simulink model "SLWF"  (R2022b)
settings: configuration reference "CommonModelConfiguration" (kept outside this file)
undefined symbols (not defined in the file): cc_param_251, LCFG_ISA_Intervention_Timeout, LCFG_ISAReactivation, LCFG_ISASoundRequest, LCFG_SLWF_Deactivation_Timeout, LCFG_VehicleBrand
settings Model: Creator=JELIASS5  LastModifiedBy=OTHOMSO1
settings ConfigSetRef: SourceName=CommonModelConfiguration  SourceLocation=Base Workspace

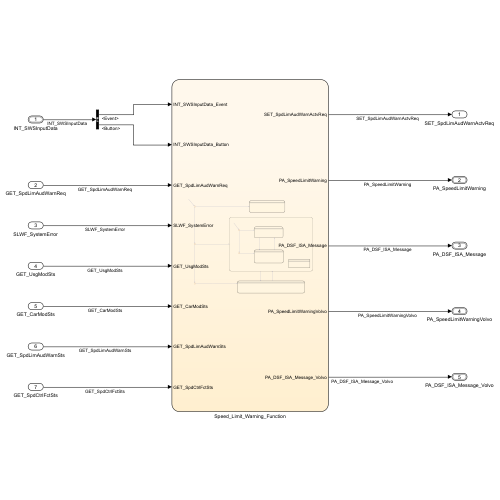
[thumbnail: Simulink's stored preview of the top-level diagram]
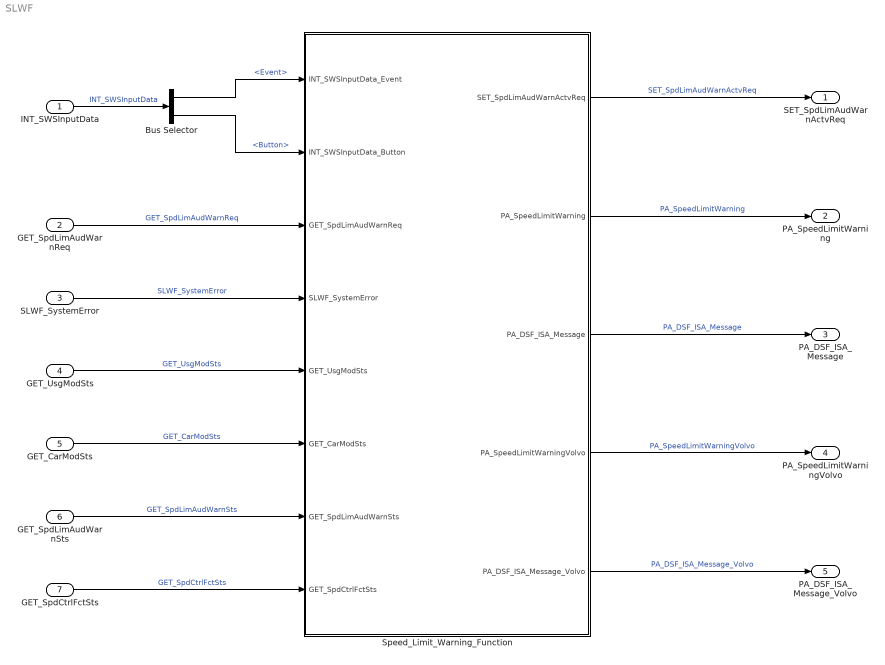
== system SLWF ==
  INT_SWSInputData : Inport  OutDataTypeStr=Bus: SWSInputData
  GET_SpdLimAudWarnReq : Inport  Port=2  OutDataTypeStr=Enum: OnOff1
  SLWF_SystemError : Inport  Port=3  OutDataTypeStr=boolean
  "GET_UsgModSts " : Inport  Port=4  OutDataTypeStr=Enum: UsgModSts1
  GET_CarModSts : Inport  Port=5  OutDataTypeStr=Enum: CarModSts1
  GET_SpdLimAudWarnSts : Inport  Port=6  OutDataTypeStr=Enum: WarnSts
  GET_SpdCtrlFctSts : Inport  Port=7  OutDataTypeStr=Enum: FctStsSpdCtrl
  Bus Selector : BusSelector  OutputSignals=Event,Button
  Speed_Limit_Warning_Function : Stateflow chart  TreatAsAtomicUnit=on
  SET_SpdLimAudWarnActvReq : Outport  OutDataTypeStr=Enum: OnOff1
  PA_SpeedLimitWarning : Outport  Port=2  OutDataTypeStr=Bus: PA_StatusAndWarningAndOffOnValue
  PA_DSF_ISA_Message : Outport  Port=3  OutDataTypeStr=Bus: PA_StatusAndOffOnValue
  PA_SpeedLimitWarningVolvo : Outport  Port=4  OutDataTypeStr=Bus: PA_StatusAndWarningAndOffOnValue
  PA_DSF_ISA_Message_Volvo : Outport  Port=5  OutDataTypeStr=Bus: PA_StatusAndOffOnValue
  wires:
  INT_SWSInputData/1 -> Bus Selector/1  "INT_SWSInputData"
  Bus Selector/1 -> Speed_Limit_Warning_Function/1(INT_SWSInputData_Event)  "<Event>"
  Bus Selector/2 -> Speed_Limit_Warning_Function/2(INT_SWSInputData_Button)  "<Button>"
  Speed_Limit_Warning_Function/1(SET_SpdLimAudWarnActvReq) -> SET_SpdLimAudWarnActvReq/1  "SET_SpdLimAudWarnActvReq"
  GET_SpdLimAudWarnReq/1 -> Speed_Limit_Warning_Function/3(GET_SpdLimAudWarnReq)  "GET_SpdLimAudWarnReq"
  Speed_Limit_Warning_Function/2(PA_SpeedLimitWarning) -> PA_SpeedLimitWarning/1  "PA_SpeedLimitWarning"
  SLWF_SystemError/1 -> Speed_Limit_Warning_Function/4(SLWF_SystemError)  "SLWF_SystemError"
  "GET_UsgModSts "/1 -> Speed_Limit_Warning_Function/5(GET_UsgModSts)  "GET_UsgModSts"
  GET_CarModSts/1 -> Speed_Limit_Warning_Function/6(GET_CarModSts)  "GET_CarModSts"
  GET_SpdLimAudWarnSts/1 -> Speed_Limit_Warning_Function/7(GET_SpdLimAudWarnSts)  "GET_SpdLimAudWarnSts"
  Speed_Limit_Warning_Function/3(PA_DSF_ISA_Message) -> PA_DSF_ISA_Message/1  "PA_DSF_ISA_Message"
  GET_SpdCtrlFctSts/1 -> Speed_Limit_Warning_Function/8(GET_SpdCtrlFctSts)  "GET_SpdCtrlFctSts"
  Speed_Limit_Warning_Function/4(PA_SpeedLimitWarningVolvo) -> PA_SpeedLimitWarningVolvo/1  "PA_SpeedLimitWarningVolvo"
  Speed_Limit_Warning_Function/5(PA_DSF_ISA_Message_Volvo) -> PA_DSF_ISA_Message_Volvo/1  "PA_DSF_ISA_Message_Volvo"

== stateflow chart SLWF/Speed_Limit_Warning_Function ==
  state CARCONFIG_INVALID
    en, du:
    SET_SpdLimAudWarnActvReq = OnOff1.OnOff1_Off;
    state CARCONFIG_INVALID_VOLVO
      en, du:
      PA_SpeedLimitWarningVolvo.Status = E_CommonStatus.NotPresent;
      PA_DSF_ISA_Message_Volvo.Status = E_CommonStatus.NotPresent;
      PA_SpeedLimitWarningVolvo.Value = E_OffOn.Off;
      PA_DSF_ISA_Message_Volvo.Value = E_OffOn.Off;
      PA_SpeedLimitWarningVolvo.Warning = E_OffOn.Off;
    state CARCONFIG_INVALID_POLESTAR
      en, du:
      PA_SpeedLimitWarning.Status = E_CommonStatus.NotPresent;
      PA_DSF_ISA_Message.Status = E_CommonStatus.NotPresent;
      PA_SpeedLimitWarning.Value = E_OffOn.Off;
      PA_DSF_ISA_Message.Value = E_OffOn.Off;
      PA_SpeedLimitWarning.Warning = E_OffOn.Off;
    (default) -> (junction 257)
    (junction 257) -> CARCONFIG_INVALID_VOLVO [order 2]
    (junction 257) -> CARCONFIG_INVALID_POLESTAR [order 1] : %Polestar
        | [LCFG_VehicleBrand == 2]
  state SYSTEM_OK
    state NOT_ACTIVE
      en, du:
      SET_SpdLimAudWarnActvReq = OnOff1.OnOff1_Off;
      state NOT_ACTIVE_VOLVO
        en, du:
        PA_SpeedLimitWarningVolvo.Status = E_CommonStatus.Disabled;
        PA_DSF_ISA_Message_Volvo.Status = E_CommonStatus.Disabled;
        PA_SpeedLimitWarningVolvo.Value = E_OffOn.Off;
        PA_DSF_ISA_Message_Volvo.Value = E_OffOn.Off;
        PA_SpeedLimitWarningVolvo.Warning = E_OffOn.Off;
      state NOT_ACTIVE_POLESTAR
        en, du:
        PA_SpeedLimitWarning.Status = E_CommonStatus.Disabled;
        PA_DSF_ISA_Message.Status = E_CommonStatus.Disabled;
        PA_SpeedLimitWarning.Value = E_OffOn.Off;
        PA_DSF_ISA_Message.Value = E_OffOn.Off;
        PA_SpeedLimitWarning.Warning = E_OffOn.Off;
      (default) -> (junction 251)
      (junction 251) -> NOT_ACTIVE_VOLVO [order 2]
      (junction 251) -> NOT_ACTIVE_POLESTAR [order 1] : %Polestar
          | [LCFG_VehicleBrand == 2]
    state ACTIVE
      state BUTTON_INTERACTION [parallel]
        settings: executionOrder=1
        state REQUEST_ON
          en, du: SET_SpdLimAudWarnActvReq = OnOff1.OnOff1_On;
        state REQUEST_OFF
          en, du: SET_SpdLimAudWarnActvReq = OnOff1.OnOff1_Off;
        (default) -> REQUEST_OFF
        REQUEST_OFF -> REQUEST_ON : %Button L2 pressed
            | [INT_SWSInputData_Button == E_SWSButton.BtnL2Req &&...
            | hasChangedTo(INT_SWSInputData_Event, E_SWSEvent.Push)]
        REQUEST_ON -> REQUEST_OFF : %Request times out
            | after(LCFG_ISASoundRequest, sec)
      state DSF_MESSAGES [parallel]
        settings: executionOrder=2
        state DSF_MESSAGE_VOLVO
          en, du:
          PA_SpeedLimitWarning.Status = E_CommonStatus.Disabled;
          PA_DSF_ISA_Message.Status = E_CommonStatus.Disabled;
          PA_SpeedLimitWarningVolvo.Status = E_CommonStatus.Available;
          PA_DSF_ISA_Message_Volvo.Status = E_CommonStatus.Available;
          state INTERVENTION
            en, du:
            PA_DSF_ISA_Message_Volvo.Value = E_OffOn.Off;
            PA_SpeedLimitWarningVolvo.Warning = E_OffOn.Off;
            PA_SpeedLimitWarningVolvo.Value = E_OffOn.On;
          state NO_MESSAGE
            en, du:
            PA_DSF_ISA_Message_Volvo.Value = E_OffOn.Off;
            PA_SpeedLimitWarningVolvo.Warning = E_OffOn.Off;
            PA_SpeedLimitWarningVolvo.Value = E_OffOn.Off;
          state MESSAGE_DISPLAYED
            en, du:
            PA_DSF_ISA_Message_Volvo.Value = E_OffOn.On;
            PA_SpeedLimitWarningVolvo.Warning = E_OffOn.On;
            PA_SpeedLimitWarningVolvo.Value = E_OffOn.Off;
          state WAIT
          state REACTIVATION_ICON
            en, du:
            PA_DSF_ISA_Message_Volvo.Value = E_OffOn.Off;
            PA_SpeedLimitWarningVolvo.Warning = E_OffOn.Off;
            PA_SpeedLimitWarningVolvo.Value = E_OffOn.On;
          (default) -> SYSTEM_OK.ACTIVE.DSF_MESSAGES.DSF_MESSAGE_VOLVO.NO_MESSAGE
          SYSTEM_OK.ACTIVE.DSF_MESSAGES.DSF_MESSAGE_VOLVO.NO_MESSAGE -> SYSTEM_OK.ACTIVE.DSF_MESSAGES.DSF_MESSAGE_VOLVO.INTERVENTION [order 3] : %Intervention from either sound or accelerator pedal response
              | [GET_SpdLimAudWarnReq == OnOff1.OnOff1_On ||...
              | GET_SpdCtrlFctSts == FctStsSpdCtrl.FctStsSpdCtrl_ActiveControlling]
          SYSTEM_OK.ACTIVE.DSF_MESSAGES.DSF_MESSAGE_VOLVO.NO_MESSAGE -> SYSTEM_OK.ACTIVE.DSF_MESSAGES.DSF_MESSAGE_VOLVO.MESSAGE_DISPLAYED [order 1] : %ISA has been turned Off
              | [hasChangedFrom(GET_SpdLimAudWarnSts, WarnSts.WarnSts_ON) &&...
              | hasChangedTo(GET_SpdLimAudWarnSts, WarnSts.WarnSts_OFF)]
          SYSTEM_OK.ACTIVE.DSF_MESSAGES.DSF_MESSAGE_VOLVO.MESSAGE_DISPLAYED -> SYSTEM_OK.ACTIVE.DSF_MESSAGES.DSF_MESSAGE_VOLVO.NO_MESSAGE [order 2] : %Timer has elapsed OR ISA has been turned On before timer has elapsed
              | [after(LCFG_SLWF_Deactivation_Timeout, sec)]
          SYSTEM_OK.ACTIVE.DSF_MESSAGES.DSF_MESSAGE_VOLVO.INTERVENTION -> SYSTEM_OK.ACTIVE.DSF_MESSAGES.DSF_MESSAGE_VOLVO.WAIT [order 1] : %Intervention stopped but shown at least LCFG time before removing it in display
              | [GET_SpdLimAudWarnReq == OnOff1.OnOff1_Off &&...
              | GET_SpdCtrlFctSts ~= FctStsSpdCtrl.FctStsSpdCtrl_ActiveControlling]
          SYSTEM_OK.ACTIVE.DSF_MESSAGES.DSF_MESSAGE_VOLVO.WAIT -> SYSTEM_OK.ACTIVE.DSF_MESSAGES.DSF_MESSAGE_VOLVO.NO_MESSAGE : [after(LCFG_ISA_Intervention_Timeout, sec)]
          SYSTEM_OK.ACTIVE.DSF_MESSAGES.DSF_MESSAGE_VOLVO.NO_MESSAGE -> SYSTEM_OK.ACTIVE.DSF_MESSAGES.DSF_MESSAGE_VOLVO.REACTIVATION_ICON [order 2] : %ISA turned on again, reactivation icon(on) displayed
              | [hasChangedFrom(GET_SpdLimAudWarnSts, WarnSts.WarnSts_OFF) &&...
              | hasChangedTo(GET_SpdLimAudWarnSts, WarnSts.WarnSts_ON)]
          SYSTEM_OK.ACTIVE.DSF_MESSAGES.DSF_MESSAGE_VOLVO.REACTIVATION_ICON -> SYSTEM_OK.ACTIVE.DSF_MESSAGES.DSF_MESSAGE_VOLVO.NO_MESSAGE [order 2] : %Reactivation icon timing out after LCFG seconds
              | [after(LCFG_ISAReactivation, sec)]
          SYSTEM_OK.ACTIVE.DSF_MESSAGES.DSF_MESSAGE_VOLVO.INTERVENTION -> SYSTEM_OK.ACTIVE.DSF_MESSAGES.DSF_MESSAGE_VOLVO.MESSAGE_DISPLAYED [order 2] : %ISA has been turned Off
              | [hasChangedFrom(GET_SpdLimAudWarnSts, WarnSts.WarnSts_ON) &&...
              | hasChangedTo(GET_SpdLimAudWarnSts, WarnSts.WarnSts_OFF)]
          SYSTEM_OK.ACTIVE.DSF_MESSAGES.DSF_MESSAGE_VOLVO.MESSAGE_DISPLAYED -> SYSTEM_OK.ACTIVE.DSF_MESSAGES.DSF_MESSAGE_VOLVO.REACTIVATION_ICON [order 1] : %ISA turned on again, reactivation icon(on) displayed
              | [hasChangedFrom(GET_SpdLimAudWarnSts, WarnSts.WarnSts_OFF) &&...
              | hasChangedTo(GET_SpdLimAudWarnSts, WarnSts.WarnSts_ON)]
          SYSTEM_OK.ACTIVE.DSF_MESSAGES.DSF_MESSAGE_VOLVO.REACTIVATION_ICON -> SYSTEM_OK.ACTIVE.DSF_MESSAGES.DSF_MESSAGE_VOLVO.MESSAGE_DISPLAYED [order 1] : %ISA has been turned Off
              | [hasChangedFrom(GET_SpdLimAudWarnSts, WarnSts.WarnSts_ON) &&...
              | hasChangedTo(GET_SpdLimAudWarnSts, WarnSts.WarnSts_OFF)]
        state DSF_MESSAGE_POLESTAR
          en, du:
          PA_SpeedLimitWarning.Status = E_CommonStatus.Available;
          PA_DSF_ISA_Message.Status = E_CommonStatus.Available;
          PA_SpeedLimitWarningVolvo.Status = E_CommonStatus.Disabled;
          PA_DSF_ISA_Message_Volvo.Status = E_CommonStatus.Disabled;
          state INTERVENTION
            en, du:
            PA_DSF_ISA_Message.Value = E_OffOn.Off;
            PA_SpeedLimitWarning.Warning = E_OffOn.Off;
            PA_SpeedLimitWarning.Value = E_OffOn.On;
          state NO_MESSAGE
            en, du:
            PA_DSF_ISA_Message.Value = E_OffOn.Off;
            PA_SpeedLimitWarning.Warning = E_OffOn.Off;
            PA_SpeedLimitWarning.Value = E_OffOn.Off;
          state MESSAGE_DISPLAYED
            en, du:
            PA_DSF_ISA_Message.Value = E_OffOn.On;
            PA_SpeedLimitWarning.Warning = E_OffOn.On;
            PA_SpeedLimitWarning.Value = E_OffOn.Off;
          state WAIT
          state REACTIVATION_ICON
            en, du:
            PA_DSF_ISA_Message.Value = E_OffOn.Off;
            PA_SpeedLimitWarning.Warning = E_OffOn.Off;
            PA_SpeedLimitWarning.Value = E_OffOn.On;
          (default) -> SYSTEM_OK.ACTIVE.DSF_MESSAGES.DSF_MESSAGE_POLESTAR.NO_MESSAGE
          SYSTEM_OK.ACTIVE.DSF_MESSAGES.DSF_MESSAGE_POLESTAR.NO_MESSAGE -> SYSTEM_OK.ACTIVE.DSF_MESSAGES.DSF_MESSAGE_POLESTAR.INTERVENTION [order 3] : %Intervention by sound
              | [GET_SpdLimAudWarnReq == OnOff1.OnOff1_On]
          SYSTEM_OK.ACTIVE.DSF_MESSAGES.DSF_MESSAGE_POLESTAR.MESSAGE_DISPLAYED -> SYSTEM_OK.ACTIVE.DSF_MESSAGES.DSF_MESSAGE_POLESTAR.NO_MESSAGE [order 2] : %Timer has elapsed, message and icon removed
              | [after(LCFG_SLWF_Deactivation_Timeout, sec)]
          SYSTEM_OK.ACTIVE.DSF_MESSAGES.DSF_MESSAGE_POLESTAR.NO_MESSAGE -> SYSTEM_OK.ACTIVE.DSF_MESSAGES.DSF_MESSAGE_POLESTAR.MESSAGE_DISPLAYED [order 1] : %ISA has been turned Off
              | [hasChangedFrom(GET_SpdLimAudWarnSts, WarnSts.WarnSts_ON) &&...
              | hasChangedTo(GET_SpdLimAudWarnSts, WarnSts.WarnSts_OFF)]
          SYSTEM_OK.ACTIVE.DSF_MESSAGES.DSF_MESSAGE_POLESTAR.WAIT -> SYSTEM_OK.ACTIVE.DSF_MESSAGES.DSF_MESSAGE_POLESTAR.NO_MESSAGE : [after(LCFG_ISA_Intervention_Timeout, sec)]
          SYSTEM_OK.ACTIVE.DSF_MESSAGES.DSF_MESSAGE_POLESTAR.INTERVENTION -> SYSTEM_OK.ACTIVE.DSF_MESSAGES.DSF_MESSAGE_POLESTAR.WAIT [order 1] : %Intervention stopped but shown at least LCFG time before removing it in display
              | [GET_SpdLimAudWarnReq == OnOff1.OnOff1_Off]
          SYSTEM_OK.ACTIVE.DSF_MESSAGES.DSF_MESSAGE_POLESTAR.NO_MESSAGE -> SYSTEM_OK.ACTIVE.DSF_MESSAGES.DSF_MESSAGE_POLESTAR.REACTIVATION_ICON [order 2] : %ISA turned on again, reactivation (on) icon displayed
              | [hasChangedFrom(GET_SpdLimAudWarnSts, WarnSts.WarnSts_OFF) &&...
              | hasChangedTo(GET_SpdLimAudWarnSts, WarnSts.WarnSts_ON)]
          SYSTEM_OK.ACTIVE.DSF_MESSAGES.DSF_MESSAGE_POLESTAR.REACTIVATION_ICON -> SYSTEM_OK.ACTIVE.DSF_MESSAGES.DSF_MESSAGE_POLESTAR.NO_MESSAGE [order 2] : %Reactivation icon timing out after LCFG seconds
              | [after(LCFG_ISAReactivation, sec)]
          SYSTEM_OK.ACTIVE.DSF_MESSAGES.DSF_MESSAGE_POLESTAR.INTERVENTION -> SYSTEM_OK.ACTIVE.DSF_MESSAGES.DSF_MESSAGE_POLESTAR.MESSAGE_DISPLAYED [order 2] : %ISA turned Off
              | [hasChangedFrom(GET_SpdLimAudWarnSts, WarnSts.WarnSts_ON) &&...
              | hasChangedTo(GET_SpdLimAudWarnSts, WarnSts.WarnSts_OFF)]
          SYSTEM_OK.ACTIVE.DSF_MESSAGES.DSF_MESSAGE_POLESTAR.MESSAGE_DISPLAYED -> SYSTEM_OK.ACTIVE.DSF_MESSAGES.DSF_MESSAGE_POLESTAR.REACTIVATION_ICON [order 1] : %ISA turned on again, reactivation icon (on) displayed
              | [hasChangedFrom(GET_SpdLimAudWarnSts, WarnSts.WarnSts_OFF) &&...
              | hasChangedTo(GET_SpdLimAudWarnSts, WarnSts.WarnSts_ON)]
          SYSTEM_OK.ACTIVE.DSF_MESSAGES.DSF_MESSAGE_POLESTAR.REACTIVATION_ICON -> SYSTEM_OK.ACTIVE.DSF_MESSAGES.DSF_MESSAGE_POLESTAR.MESSAGE_DISPLAYED [order 1] : %ISA has been turned off
              | [hasChangedFrom(GET_SpdLimAudWarnSts, WarnSts.WarnSts_ON) &&...
              | hasChangedTo(GET_SpdLimAudWarnSts, WarnSts.WarnSts_OFF)]
        (default) -> (junction 164)
        (junction 164) -> DSF_MESSAGE_VOLVO [order 2]
        (junction 164) -> DSF_MESSAGE_POLESTAR [order 1] : %Polestar
            | [LCFG_VehicleBrand == 2]
    state isActive = activationCheck [function]
      (default) -> (junction 42)
      (junction 42) -> (junction 46) [order 1] : [GET_UsgModSts == UsgModSts1.UsgModSts1_UsgModDrvg &&...
          | GET_CarModSts == CarModSts1.CarModSts1_CarModNorm]
      (junction 42) -> (junction 47) [order 2] : {isActive = false;}
      (junction 46) -> (junction 48) : {isActive = true;}
      (junction 48) -> (junction 47)
      (junction 47) -> (junction 49)
    (default) -> (junction 30)
    (junction 30) -> NOT_ACTIVE [order 1] : [~activationCheck()]
    (junction 30) -> (junction 33) [order 2]
    NOT_ACTIVE -> ACTIVE : [activationCheck()]
    ACTIVE -> NOT_ACTIVE : [~activationCheck()]
    (junction 33) -> ACTIVE
  state SYSTEM_ERROR
    en, du:
    SET_SpdLimAudWarnActvReq = OnOff1.OnOff1_Off;
    state SYSTEM_ERROR_VOLVO
      en, du:
      PA_SpeedLimitWarningVolvo.Status = E_CommonStatus.SystemError;
      PA_DSF_ISA_Message_Volvo.Status = E_CommonStatus.SystemError;
      PA_SpeedLimitWarningVolvo.Value = E_OffOn.Off;
      PA_DSF_ISA_Message_Volvo.Value = E_OffOn.Off;
      PA_SpeedLimitWarningVolvo.Warning = E_OffOn.Off;
    state SYSTEM_ERROR_POLESTAR
      en, du:
      PA_SpeedLimitWarning.Status = E_CommonStatus.SystemError;
      PA_DSF_ISA_Message.Status = E_CommonStatus.SystemError;
      PA_SpeedLimitWarning.Value = E_OffOn.Off;
      PA_DSF_ISA_Message.Value = E_OffOn.Off;
      PA_SpeedLimitWarning.Warning = E_OffOn.Off;
    (default) -> (junction 245)
    (junction 245) -> SYSTEM_ERROR_POLESTAR [order 1] : %Polestar
        | [LCFG_VehicleBrand == 2]
    (junction 245) -> SYSTEM_ERROR_VOLVO [order 2]
  (default) -> (junction 14)
  (junction 14) -> CARCONFIG_INVALID [order 2]
  (junction 14) -> (junction 17) [order 1] : [(cc_param_251 == 2||...
      | cc_param_251 == 3)]
  (junction 17) -> SYSTEM_OK [order 1] : [SLWF_SystemError == false]
  (junction 17) -> (junction 20) [order 2]
  SYSTEM_OK -> SYSTEM_ERROR : [SLWF_SystemError == true]
  SYSTEM_ERROR -> SYSTEM_OK : [SLWF_SystemError == false]
  (junction 20) -> SYSTEM_ERROR
  data: isActive function_output; INT_SWSInputData_Event input Enum: E_SWSEvent; INT_SWSInputData_Button input Enum: E_SWSButton; SET_SpdLimAudWarnActvReq output Enum: OnOff1; PA_SpeedLimitWarning output Bus: PA_StatusAndWarningAndOffOnValue; cc_param_251 parameter uint8; GET_SpdLimAudWarnReq input Enum: OnOff1; SLWF_SystemError input boolean; GET_UsgModSts input Enum: UsgModSts1; GET_CarModSts input Enum: CarModSts1; LCFG_ISASoundRequest parameter single; GET_SpdLimAudWarnSts input Enum: WarnSts; PA_DSF_ISA_Message output Bus: PA_StatusAndOffOnValue; LCFG_SLWF_Deactivation_Timeout parameter single; GET_SpdCtrlFctSts input Enum: FctStsSpdCtrl; LCFG_VehicleBrand parameter single; PA_SpeedLimitWarningVolvo output Bus: PA_StatusAndWarningAndOffOnValue; PA_DSF_ISA_Message_Volvo output Bus: PA_StatusAndOffOnValue; LCFG_ISAReactivation parameter single; LCFG_ISA_Intervention_Timeout parameter single
